simulink model "MicroMouseTemplate"  (R2023a)
settings: Solver=FixedStepAuto  StartTime=0.0  StopTime=10.0  RelTol=1e-3
values from neighbouring files (symbols this model uses):
  IR_LED_PERIOD = 0.05    [runMeFirst.m]
  signalWindowLength = 20    [runMeFirst.m]
  TIM3_ARR = 4000    [runMeFirst.m]
undefined symbols (not defined in the file or in its folder): ADC_H, ADC_L
libraries: dspstat3 x36, stm32f4xxblockslib x16, stm32l4xxblockslib x4, stm32blockslib x1
settings Model: Creator=JesseJabezArendse  LastModifiedBy=JesseJabezArendse
settings SolverCC: AllowMultiTaskInputOutput=on  InsertRTBMode=Never (minimum delay)
settings OptimizationCC: EnhancedBackFolding=on  PassReuseOutputArgsAs=Individual arguments  ZeroExternalMemoryAtStartup=off  ZeroInternalMemoryAtStartup=off  MaxStackSize=64  OptimizeBlockOrder=speed  DifferentSizesBufferReuse=on  OptimizationCustomize=off  EfficientTunableParamExpr=on
settings DebuggingCC: MultiTaskCondExecSysMsg=none  ParameterOverflowMsg=none  ParameterPrecisionLossMsg=none  ParameterTunabilityLossMsg=error
settings HardwareCC: ProdBitPerPointer=32  ProdBitPerSizeT=32  ProdBitPerPtrDiffT=32  ProdLargestAtomicInteger=Long  ProdLargestAtomicFloat=Double  ProdWordSize=32  ProdLongLongMode=on  ProdHWDeviceType=ARM Compatible->ARM Cortex
settings ModelReferenceCC: EnableParallelModelReferenceBuilds=on
settings SFSimCC: MATLABDynamicMemAlloc=off
settings RTWCC: Description=Embedded Coder  SystemTargetFile=ert.tlc  HardwareBoard=STM32L4xx Based  TemplateMakefile=ert_default_tmf  Toolchain=GNU Tools for ARM Embedded Processors
settings RTWCC: CustomHeaderCode=|
  | #include "MicroMouseProgramming\Core\Inc\IMU.h"
  | #include "MicroMouseProgramming\Core\Inc\CustomWhile.h"
  | #include "MicroMouseProgramming\Core\Inc\Motors.h"
settings RTWCC: CustomInclude=|
  | MicroMouseProgramming\Core\Inc\
  | MicroMouseProgramming\Core\Src\
settings RTWCC: CustomSource=|
  | MicroMouseProgramming\Core\Src\IMU.c
  | MicroMouseProgramming\Core\Src\CustomWhile.c
  | MicroMouseProgramming\Core\Src\Motors.c
settings CodeAppCC: ForceParamTrailComments=on  IgnoreCustomStorageClasses=off  OperatorAnnotations=on  SimulinkDataObjDesc=on  SFDataObjDesc=on  InsertBlockDesc=on
settings ERTTargetCC: CodeReplacementLibrary=ARM Cortex-M  SupportContinuousTime=on  ExtModeTransport=3  ExtModeStaticAlloc=on  ExtModeStaticAllocSize=2048  ExtModeMexFile=ext_xcp  ExtModeIntrfLevel=Level2 - Open

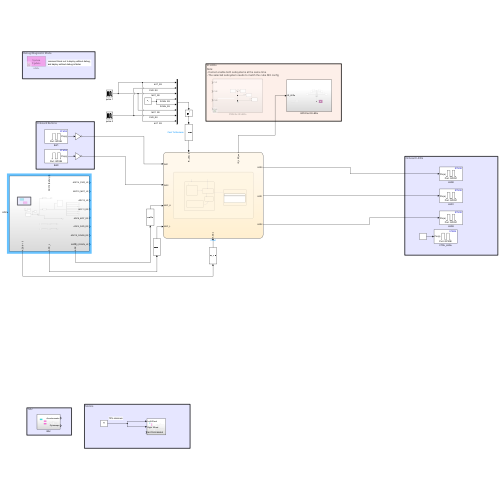
[thumbnail: Simulink's stored preview of the top-level diagram]
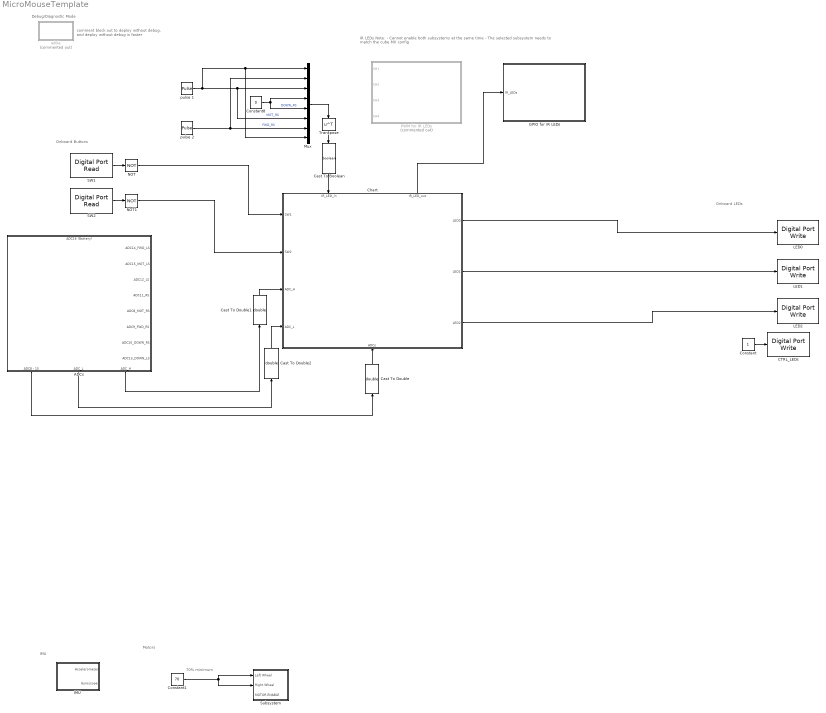
== system MicroMouseTemplate ==
  note: 70% minimum
  note: Motors
  note: IR LEDs
      | Note:
      | - Cannot enable both subsystems at the same time
      | - The selected subsystem needs to match the cube MX config
  note: IMU
  note: Onboard Buttons
  note: comment block out to deploy without debug, and deploy without debug is faster
  note: Onboard LEDs
  note: Debug/Diagnostic Mode
  "ADCs " : Subsystem
      settings: PortSchema="{\"entries\":[{\"content\":{\"sides\":[{\"content\":{},\"type\":\"ConnectorPlacement.EquallySpacedRectSide\",\"uuid\":\"ad9b4559-80f4-4a8a-ae53-5c16a02c7140\"},{\"content\":{\"connectorIds\":[\"Out1\",\"Out2\",\"Out3\",\"Out4\",\"Out5\",\"Out6\",\"Out7\",\"Out8\"],\"side\":\"RIGHT\"},\"type\":\"ConnectorPlacement.EquallySpacedRectSide\",\"uuid\":\"bb9b2394-70a2-4e95-b5de-6e9e6d3444df\"},{\"content\":{\"connectorIds\":[\"Out12\"],\"side\":\"TOP\"},\"type\":\"ConnectorPlacement.EquallySpacedRectSide\",\"uuid\":\"a0caae28-44ef-4496-b197-488b1b027954\"},{\"content\":{\"connectorIds\":[\"Out9\",\"Out10\",\"Out11\"],\"side\":\"BOTTOM\"},\"type\":\"ConnectorPlacement.EquallySpacedRectSide\",\"uuid\":\"aca5f2a6-b788-4b53-b626-f7b89ca7e1d4\"}]},\"type\":\"ConnectorPlacement.EquallySpacedConnector\",\"uuid\":\"1ade7d4f-8aae-4b0d-9bfd-23fa99654b08\"}],\"packageUris\":[\"http://schema.mathworks.com/mf0/Connector/R2020b\"],\"version\":\"1.0\"}"
  CTRL_LEDs : stm32f4xxblockslib/Digital Port Write  PortName=GPIOB  PinNumber=3  ReadOperation=off  IOAsArray=on  EnableSimPort=off
      settings: LibrarySourceBlock=stm32l4xxblockslib/Digital Port Write
  Cast To Boolean : DataTypeConversion  OutDataTypeStr=boolean  SaturateOnIntegerOverflow=off  RndMeth=Floor
  Cast To Double : DataTypeConversion  OutDataTypeStr=double  SaturateOnIntegerOverflow=off  RndMeth=Floor
  Cast To Double1 : DataTypeConversion  OutDataTypeStr=double  SaturateOnIntegerOverflow=off  RndMeth=Floor
  Cast To Double2 : DataTypeConversion  OutDataTypeStr=double  SaturateOnIntegerOverflow=off  RndMeth=Floor
  Chart : Stateflow chart  TreatAsAtomicUnit=on
      settings: PortSchema="{\"entries\":[{\"content\":{\"sides\":[{\"content\":{\"connectorIds\":[\"In2\",\"In3\",\"In4\",\"In5\"]},\"type\":\"ConnectorPlacement.EquallySpacedRectSide\",\"uuid\":\"32f6fed0-3232-4bab-b39d-a3af84b75639\"},{\"content\":{\"connectorIds\":[\"Out1\",\"Out2\",\"Out3\"],\"side\":\"RIGHT\"},\"type\":\"ConnectorPlacement.EquallySpacedRectSide\",\"uuid\":\"0c32a1fe-915a-4e8a-b3ee-800457e23572\"},{\"content\":{\"connectorIds\":[\"In6\",\"Out4\"],\"side\":\"TOP\"},\"type\":\"ConnectorPlacement.EquallySpacedRectSide\",\"uuid\":\"1ac04b60-bb97-4700-a588-8796c93b1b04\"},{\"content\":{\"connectorIds\":[\"In1\"],\"side\":\"BOTTOM\"},\"type\":\"ConnectorPlacement.EquallySpacedRectSide\",\"uuid\":\"5382ec1b-aa52-4e38-a7ba-82e952b8f427\"}]},\"type\":\"ConnectorPlacement.EquallySpacedConnector\",\"uuid\":\"e2f36b59-a9e2-4f43-a02a-04bcc2f7ebe2\"}],\"packageUris\":[\"http://schema.mathworks.com/mf0/Connector/R2020b\"],\"version\":\"1.0\"}"
  Constant : Constant
  Constant1 : Constant  Value=70
  Constant8 : Constant  Value=0
  GPIO for IR LEDs : Subsystem
  IMU : Subsystem
  LED0 : stm32f4xxblockslib/Digital Port Write  PortName=GPIOC  PinNumber=[13]  ReadOperation=off  IOAsArray=on  EnableSimPort=off
      settings: LibrarySourceBlock=stm32l4xxblockslib/Digital Port Write
  LED1 : stm32f4xxblockslib/Digital Port Write  PortName=GPIOC  PinNumber=[14]  ReadOperation=off  IOAsArray=on  EnableSimPort=off
      settings: LibrarySourceBlock=stm32l4xxblockslib/Digital Port Write
  LED2 : stm32f4xxblockslib/Digital Port Write  PortName=GPIOC  PinNumber=[15]  ReadOperation=off  IOAsArray=on  EnableSimPort=off
      settings: LibrarySourceBlock=stm32l4xxblockslib/Digital Port Write
  Mux : Mux  Inputs=8
  NOT : Logic  Operator=NOT  IconShape=distinctive  AllPortsSameDT=off  OutDataTypeStr=boolean
  NOT1 : Logic  Operator=NOT  IconShape=distinctive  AllPortsSameDT=off  OutDataTypeStr=boolean
  "PWM for IR LEDs " : Subsystem  Commented=on
  SW1 : stm32f4xxblockslib/Digital Port Read  PortName=GPIOE  PinNumber=[6]  ReadOperation=on  IOAsArray=on  SampleTime=-1  EnableSimPort=off
      settings: LibrarySourceBlock=stm32l4xxblockslib/Digital Port Read
  SW2 : stm32f4xxblockslib/Digital Port Read  PortName=GPIOB  PinNumber=[2]  ReadOperation=on  IOAsArray=on  SampleTime=-1  EnableSimPort=off
      settings: LibrarySourceBlock=stm32l4xxblockslib/Digital Port Read
  Subsystem : Subsystem
  Transpose : Math  Operator=transpose
  pulse 1 : DiscretePulseGenerator  PulseType=Time based  Period=3*IR_LED_PERIOD  PulseWidth=1/4*100
  pulse 2 : DiscretePulseGenerator  PulseType=Time based  Period=3*IR_LED_PERIOD  PulseWidth=1/4*100  PhaseDelay=2*IR_LED_PERIOD
  while : Subsystem  Commented=on  mask(System Update){ShowInLibBrowser=0}
      mask prompts: ShowInLibBrowser "Simulink:masks:CustCodeMaskParam1_MP"
      settings: CopyFcn=cccopyfcn(gcb)  OpenFcn=ccopenfcn('System Update Function')
      mask Help: eval('feval(''rtwprivate'',''rtwhelpview'',''rtw_sys_update_block'')');
      mask DialogControl ShowInLibBrowser Prompt: Mask Parameter 1:
      mask Display: disp('System\nUpdate');
  wires:
  SW2/1 -> NOT1/1
  Constant/1 -> CTRL_LEDs/1
  SW1/1 -> NOT/1
  Constant1/1 -> Subsystem/1(Left Wheel), Subsystem/2(Right Wheel)
  pulse 2/1 -> Mux/2, Mux/7  "FWD_RS"
  pulse 1/1 -> Mux/8, Mux/1, Mux/6, Mux/3  "MOT_RS"
  Constant8/1 -> Mux/4, Mux/5  "DOWN_RS"
  Mux/1 -> Transpose/1
  Chart/1(LED0) -> LED0/1
  Chart/2(LED1) -> LED1/1
  Chart/3(LED2) -> LED2/1
  "ADCs "/11(ADC_H) -> Cast To Double1/1
  "ADCs "/10(ADC_L) -> Cast To Double2/1
  Chart/4(IR_LED_out) -> GPIO for IR LEDs/1(IR_LEDs)
  NOT/1 -> Chart/2(SW1)
  NOT1/1 -> Chart/3(SW2)
  Transpose/1 -> Cast To Boolean/1
  Cast To Boolean/1 -> Chart/6(IR_LED_in)
  "ADCs "/9(ADC8 - 15) -> Cast To Double/1
  Cast To Double/1 -> Chart/1(ADCs)
  Cast To Double1/1 -> Chart/4(ADC_H)
  Cast To Double2/1 -> Chart/5(ADC_L)

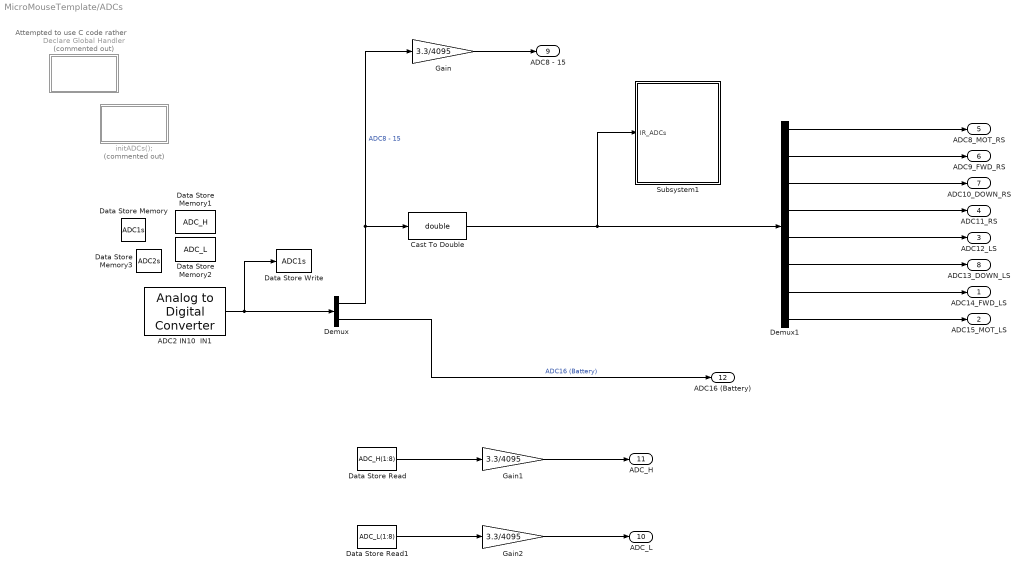
== system MicroMouseTemplate/ADCs  ==
  note: Attempted to use C code rather
  ADC2 IN10  IN1 : stm32f4xxblockslib/Analog to Digital Converter  ADCModule=ADC2  ConversionGroup=Regular  TriggerMode=Trigger and read  NumberOfConversions=9  EnableBufferConv=on  BufferLength=9  OutputStatus=off  SampleTime=-1  EnableSimPort=off
      settings: LibrarySourceBlock=stm32l4xxblockslib/Analog to Digital Converter
  Cast To Double : DataTypeConversion  OutDataTypeStr=double  SaturateOnIntegerOverflow=off  RndMeth=Floor
  Data Store Memory : DataStoreMemory  DataStoreName=ADC1s  WriteAfterWriteMsg=warning  ShowAdditionalParam=off  OutDataTypeStr=uint16  Dimensions=9
  Data Store Memory1 : DataStoreMemory  DataStoreName=ADC_H  WriteAfterWriteMsg=warning  ShowAdditionalParam=off  OutDataTypeStr=uint16  Dimensions=9
  Data Store Memory2 : DataStoreMemory  DataStoreName=ADC_L  WriteAfterWriteMsg=warning  ShowAdditionalParam=off  OutDataTypeStr=uint16  Dimensions=9
  Data Store Memory3 : DataStoreMemory  DataStoreName=ADC2s  WriteAfterWriteMsg=warning  ShowAdditionalParam=off  OutDataTypeStr=uint16  Dimensions=9
  Data Store Read : DataStoreRead  DataStoreName=ADC_H  DataStoreElements=ADC_H(1:8)  NumberOfDimensions=8  IndexOptions=Index vector (dialog),Index vector (dialog),Index vector (dialog),Index vector (dialog),Index vector (dialog),Index vector (dialog),Index vector (dialog),Index vector (dialog)  Indices=1,1,1,1,1,1,1,1  OutputSizes=1,1,1,1,1,1,1,1
  Data Store Read1 : DataStoreRead  DataStoreName=ADC_L  DataStoreElements=ADC_L(1:8)  IndexOptions=Index vector (dialog)  Indices=1  OutputSizes=1
  Data Store Write : DataStoreWrite  DataStoreName=ADC1s  IndexOptions=Index vector (dialog)  Indices=1  OutputSizes=1
  Declare Global Handler : Subsystem  Commented=on  mask(Model Source){ShowInLibBrowser=0}
      mask prompts: ShowInLibBrowser "Simulink:masks:CustCodeMaskParam1_MP"
      settings: CopyFcn=cccopyfcn(gcb)  OpenFcn=ccopenfcn('Model Source')
      mask Help: eval('feval(''rtwprivate'',''rtwhelpview'',''rtw_model_source_block'')');
      mask Display: disp('Model\nSource');
  Demux : Demux  Outputs=[8 1]
  Demux1 : Demux  Outputs=8
  Gain : Gain  Gain=3.3/4095
  Gain1 : Gain  Gain=3.3/4095
  Gain2 : Gain  Gain=3.3/4095
  Subsystem1 : Subsystem
  initADCs(); : Subsystem  Commented=on  mask(System Initialize){ShowInLibBrowser=0}
      mask prompts: ShowInLibBrowser "Simulink:masks:CustCodeMaskParam1_MP"
      settings: CopyFcn=cccopyfcn(gcb)  OpenFcn=ccopenfcn('System Initialize Function')
      mask Help: eval('feval(''rtwprivate'',''rtwhelpview'',''rtw_sys_initialize_block'')');
      mask Display: disp('System\nInitialize');
  ADC14_FWD_LS : Outport
  ADC15_MOT_LS : Outport  Port=2
  ADC12_LS : Outport  Port=3
  ADC11_RS : Outport  Port=4
  ADC8_MOT_RS : Outport  Port=5
  ADC9_FWD_RS : Outport  Port=6
  ADC10_DOWN_RS : Outport  Port=7
  ADC13_DOWN_LS : Outport  Port=8
  ADC8 - 15 : Outport  Port=9
  ADC_L : Outport  Port=10
  ADC_H : Outport  Port=11
  ADC16 (Battery) : Outport  Port=12
  wires:
  Demux/1 -> Gain/1, Cast To Double/1  "ADC8 - 15"
  Demux/2 -> ADC16 (Battery)/1  "ADC16 (Battery)"
  Demux1/1 -> ADC8_MOT_RS/1
  Demux1/2 -> ADC9_FWD_RS/1
  Demux1/3 -> ADC10_DOWN_RS/1
  Demux1/4 -> ADC11_RS/1
  Demux1/5 -> ADC12_LS/1
  Demux1/6 -> ADC13_DOWN_LS/1
  Demux1/7 -> ADC14_FWD_LS/1
  Demux1/8 -> ADC15_MOT_LS/1
  ADC2 IN10  IN1/1 -> Data Store Write/1, Demux/1
  Cast To Double/1 -> Demux1/1, Subsystem1/1(IR_ADCs)
  Gain/1 -> ADC8 - 15/1
  Data Store Read/1 -> Gain1/1
  Data Store Read1/1 -> Gain2/1
  Gain1/1 -> ADC_H/1
  Gain2/1 -> ADC_L/1

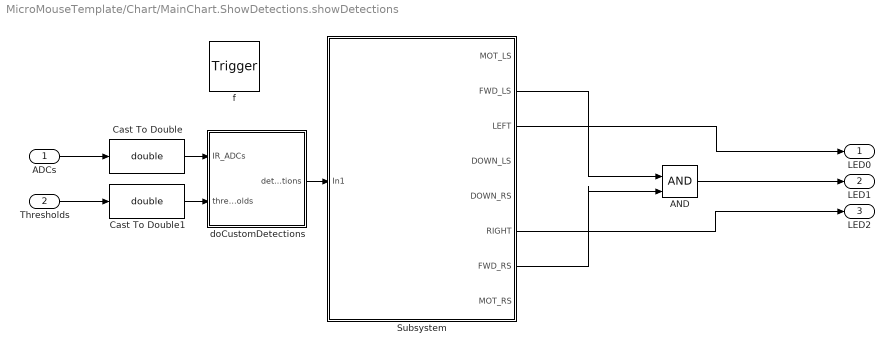
== system MicroMouseTemplate/Chart/MainChart.ShowDetections.showDetections ==
  ADCs : Inport  OutDataTypeStr=double  PortDimensions=8
  Thresholds : Inport  Port=2  OutDataTypeStr=double  PortDimensions=8
  f : TriggerPort  TriggerType=function-call  VariantControl=(inherit)
      settings: CopyFcn=Stateflow.SLINSF.SimulinkMan.removeBlockPreDeleteFcn  PreDeleteFcn=Stateflow.SLINSF.SimulinkMan.unsafePredeleteFcn
  AND : Logic  IconShape=distinctive  AllPortsSameDT=off  OutDataTypeStr=boolean
  Cast To Double : DataTypeConversion  OutDataTypeStr=double  SaturateOnIntegerOverflow=off  RndMeth=Floor
  Cast To Double1 : DataTypeConversion  OutDataTypeStr=double  SaturateOnIntegerOverflow=off  RndMeth=Floor
  Subsystem : Subsystem
  doCustomDetections : Subsystem
  LED0 : Outport
  LED1 : Outport  Port=2
  LED2 : Outport  Port=3
  wires:
  Subsystem/7(FWD_RS) -> AND/2
  AND/1 -> LED1/1
  Subsystem/2(FWD_LS) -> AND/1
  Subsystem/3(LEFT) -> LED0/1
  Subsystem/6(RIGHT) -> LED2/1
  ADCs/1 -> Cast To Double/1
  Thresholds/1 -> Cast To Double1/1
  doCustomDetections/1(detections) -> Subsystem/1(In1)
  Cast To Double/1 -> doCustomDetections/1(IR_ADCs)
  Cast To Double1/1 -> doCustomDetections/2(thresholds)

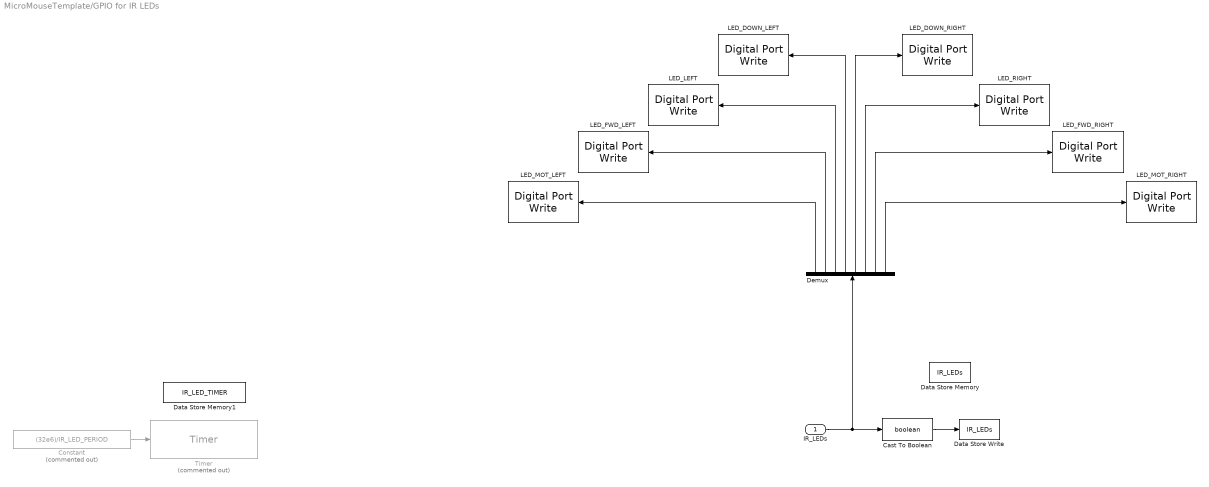
== system MicroMouseTemplate/GPIO for IR LEDs ==
  IR_LEDs : Inport
  Cast To Boolean : DataTypeConversion  OutDataTypeStr=boolean  SaturateOnIntegerOverflow=off  RndMeth=Floor
  Constant : Constant  Commented=on  Value=(32e6)/IR_LED_PERIOD
  Data Store Memory : DataStoreMemory  DataStoreName=IR_LEDs  WriteAfterWriteMsg=warning  ShowAdditionalParam=off  OutDataTypeStr=boolean  Dimensions=8
  Data Store Memory1 : DataStoreMemory  DataStoreName=IR_LED_TIMER  WriteAfterWriteMsg=warning  ShowAdditionalParam=off  OutDataTypeStr=uint32  Dimensions=1
  Data Store Write : DataStoreWrite  DataStoreName=IR_LEDs  IndexOptions=Index vector (dialog)  Indices=1  OutputSizes=1
  Demux : Demux  Outputs=8
  LED_DOWN_LEFT : stm32f4xxblockslib/Digital Port Write  PortName=GPIOE  PinNumber=9  ReadOperation=off  IOAsArray=on  EnableSimPort=off
      settings: LibrarySourceBlock=stm32l4xxblockslib/Digital Port Write
  LED_DOWN_RIGHT : stm32f4xxblockslib/Digital Port Write  PortName=GPIOE  PinNumber=14  ReadOperation=off  IOAsArray=on  EnableSimPort=off
      settings: LibrarySourceBlock=stm32l4xxblockslib/Digital Port Write
  LED_FWD_LEFT : stm32f4xxblockslib/Digital Port Write  PortName=GPIOE  PinNumber=8  ReadOperation=off  IOAsArray=on  EnableSimPort=off
      settings: LibrarySourceBlock=stm32l4xxblockslib/Digital Port Write
  LED_FWD_RIGHT : stm32f4xxblockslib/Digital Port Write  PortName=GPIOE  PinNumber=15  ReadOperation=off  IOAsArray=on  EnableSimPort=off
      settings: LibrarySourceBlock=stm32l4xxblockslib/Digital Port Write
  LED_LEFT : stm32f4xxblockslib/Digital Port Write  PortName=GPIOE  PinNumber=12  ReadOperation=off  IOAsArray=on  EnableSimPort=off
      settings: LibrarySourceBlock=stm32l4xxblockslib/Digital Port Write
  LED_MOT_LEFT : stm32f4xxblockslib/Digital Port Write  PortName=GPIOB  PinNumber=12  ReadOperation=off  IOAsArray=on  EnableSimPort=off
      settings: LibrarySourceBlock=stm32l4xxblockslib/Digital Port Write
  LED_MOT_RIGHT : stm32f4xxblockslib/Digital Port Write  PortName=GPIOE  PinNumber=13  ReadOperation=off  IOAsArray=on  EnableSimPort=off
      settings: LibrarySourceBlock=stm32l4xxblockslib/Digital Port Write
  LED_RIGHT : stm32f4xxblockslib/Digital Port Write  PortName=GPIOE  PinNumber=11  ReadOperation=off  IOAsArray=on  EnableSimPort=off
      settings: LibrarySourceBlock=stm32l4xxblockslib/Digital Port Write
  Timer : stm32blockslib/Timer  Priority=4  Commented=on  TimerModule=TIM4  EnableFrequencyInput=on  EnableCounterInput=off  EnableMainOutputInput=off  SetRCAfterCE=off  OutputDirection=off  OutputMainOutputEnableStatus=off  SampleTime=-1  EnableUpdateEvent=off  EnableCaptureCompare1Event=off  EnableCaptureCompare2Event=off  EnableCaptureCompare3Event=off  EnableCaptureCompare4Event=off  EnableTriggerEvent=off  EnableBreakEvent=off  EnableBreakEvent2=off  EnableCOMGenerationEvent=off  ProcessorFamily=STM32L4
      settings: LibrarySourceBlock=stm32l4xxblockslib/Timer
  wires:
  Demux/1 -> LED_MOT_LEFT/1
  Demux/2 -> LED_FWD_LEFT/1
  Demux/3 -> LED_LEFT/1
  Constant/1 -> Timer/1
  IR_LEDs/1 -> Demux/1, Cast To Boolean/1
  Demux/6 -> LED_RIGHT/1
  Demux/7 -> LED_FWD_RIGHT/1
  Demux/8 -> LED_MOT_RIGHT/1
  Demux/4 -> LED_DOWN_LEFT/1
  Demux/5 -> LED_DOWN_RIGHT/1
  Cast To Boolean/1 -> Data Store Write/1

== system MicroMouseTemplate/IMU ==
  Data Store Memory : DataStoreMemory  DataStoreName=IMU_Accel  WriteAfterWriteMsg=warning  ShowAdditionalParam=off  OutDataTypeStr=single  Dimensions=3
  Data Store Memory1 : DataStoreMemory  DataStoreName=IMU_Gyro  WriteAfterWriteMsg=warning  ShowAdditionalParam=off  OutDataTypeStr=single  Dimensions=3
  Data Store Read : DataStoreRead  DataStoreName=IMU_Accel  IndexOptions=Index vector (dialog)  Indices=1  OutputSizes=1
  Data Store Read1 : DataStoreRead  DataStoreName=IMU_Gyro  IndexOptions=Index vector (dialog)  Indices=1  OutputSizes=1
  Declare Global Handler : Subsystem  mask(Model Source){ShowInLibBrowser=0}
      mask prompts: ShowInLibBrowser "Simulink:masks:CustCodeMaskParam1_MP"
      settings: CopyFcn=cccopyfcn(gcb)  OpenFcn=ccopenfcn('Model Source')
      mask Help: eval('feval(''rtwprivate'',''rtwhelpview'',''rtw_model_source_block'')');
      mask Display: disp('Model\nSource');
  initIMU(); : Subsystem  mask(System Initialize){ShowInLibBrowser=0}
      mask prompts: ShowInLibBrowser "Simulink:masks:CustCodeMaskParam1_MP"
      settings: CopyFcn=cccopyfcn(gcb)  OpenFcn=ccopenfcn('System Initialize Function')
      mask Help: eval('feval(''rtwprivate'',''rtwhelpview'',''rtw_sys_initialize_block'')');
      mask Display: disp('System\nInitialize');
  refreshIMUValues(); : Subsystem  mask(System Update){ShowInLibBrowser=0}
      mask prompts: ShowInLibBrowser "Simulink:masks:CustCodeMaskParam1_MP"
      settings: CopyFcn=cccopyfcn(gcb)  OpenFcn=ccopenfcn('System Update Function')
      mask Help: eval('feval(''rtwprivate'',''rtwhelpview'',''rtw_sys_update_block'')');
      mask Display: disp('System\nUpdate');
  Accelerometer : Outport
  Gyroscope : Outport  Port=2
  wires:
  Data Store Read1/1 -> Gyroscope/1
  Data Store Read/1 -> Accelerometer/1

== system MicroMouseTemplate/PWM for IR LEDs  ==
  note: the others are not availible, either a negative channel or not a PWM pin
  CH1 : Inport
  CH2 : Inport  Port=2
  CH3 : Inport  Port=3
  CH4 : Inport  Port=4
  ENABLE PWM MODE : Constant  Value=0
  LED_PWM_FWD_RIGHT : stm32l4xxblockslib/PWM Output  TimerModule=TIM1  DutycycleUnits=Percentage  EnableChannel1=off  EnableChannel2=off  EnableChannel3=on  EnableChannel4=off  EnableChannel5=off  EnableChannel6=off  EnableCounterInput=on  EnableMainOutputInput=off  EnableFrequencyInput=off  SetRCAfterCE=off  OutputDirection=off  OutputMainOutputEnableStatus=off  SampleTime=0.1  EnableSimPort=off  EnableUpdateEvent=off  EnableCaptureCompare1Event=off  EnableCaptureCompare2Event=off  EnableCaptureCompare3Event=off  EnableCaptureCompare4Event=off  EnableTriggerEvent=off  EnableBreakEvent=off  EnableBreakEvent2=off  ProcessorFamily=STM32L4  hoistedMaskSrc=ECSoC/ECSimCodegen/PWM Output
  LED_PWM_LEFT : stm32l4xxblockslib/PWM Output  TimerModule=TIM1  DutycycleUnits=Percentage  EnableChannel1=on  EnableChannel2=off  EnableChannel3=off  EnableChannel4=off  EnableChannel5=off  EnableChannel6=off  EnableCounterInput=on  EnableMainOutputInput=off  EnableFrequencyInput=off  SetRCAfterCE=off  OutputDirection=off  OutputMainOutputEnableStatus=off  SampleTime=0.1  EnableSimPort=off  EnableUpdateEvent=off  EnableCaptureCompare1Event=off  EnableCaptureCompare2Event=off  EnableCaptureCompare3Event=off  EnableCaptureCompare4Event=off  EnableTriggerEvent=off  EnableBreakEvent=off  EnableBreakEvent2=off  ProcessorFamily=STM32L4  hoistedMaskSrc=ECSoC/ECSimCodegen/PWM Output
  LED_PWM_MOT_RIGHT : stm32l4xxblockslib/PWM Output  TimerModule=TIM17  DutycycleUnits=Percentage  EnableChannel1=on  EnableChannel2=off  EnableChannel3=off  EnableChannel4=off  EnableChannel5=off  EnableChannel6=off  EnableCounterInput=on  EnableMainOutputInput=off  EnableFrequencyInput=off  SetRCAfterCE=off  OutputDirection=off  OutputMainOutputEnableStatus=off  SampleTime=0.1  EnableSimPort=off  EnableUpdateEvent=off  EnableCaptureCompare1Event=off  EnableCaptureCompare2Event=off  EnableCaptureCompare3Event=off  EnableCaptureCompare4Event=off  EnableTriggerEvent=off  EnableBreakEvent=off  EnableBreakEvent2=off  ProcessorFamily=STM32L4  hoistedMaskSrc=ECSoC/ECSimCodegen/PWM Output
  LED_PWM_RIGHT : stm32l4xxblockslib/PWM Output  TimerModule=TIM1  DutycycleUnits=Percentage  EnableChannel1=off  EnableChannel2=on  EnableChannel3=off  EnableChannel4=off  EnableChannel5=off  EnableChannel6=off  EnableCounterInput=on  EnableMainOutputInput=off  EnableFrequencyInput=off  SetRCAfterCE=off  OutputDirection=off  OutputMainOutputEnableStatus=off  SampleTime=0.1  EnableSimPort=off  EnableUpdateEvent=off  EnableCaptureCompare1Event=off  EnableCaptureCompare2Event=off  EnableCaptureCompare3Event=off  EnableCaptureCompare4Event=off  EnableTriggerEvent=off  EnableBreakEvent=off  EnableBreakEvent2=off  ProcessorFamily=STM32L4  hoistedMaskSrc=ECSoC/ECSimCodegen/PWM Output
  wires:
  ENABLE PWM MODE/1 -> LED_PWM_RIGHT/2, LED_PWM_LEFT/2, LED_PWM_FWD_RIGHT/2, LED_PWM_MOT_RIGHT/2
  CH1/1 -> LED_PWM_LEFT/1
  CH4/1 -> LED_PWM_MOT_RIGHT/1
  CH2/1 -> LED_PWM_RIGHT/1
  CH3/1 -> LED_PWM_FWD_RIGHT/1

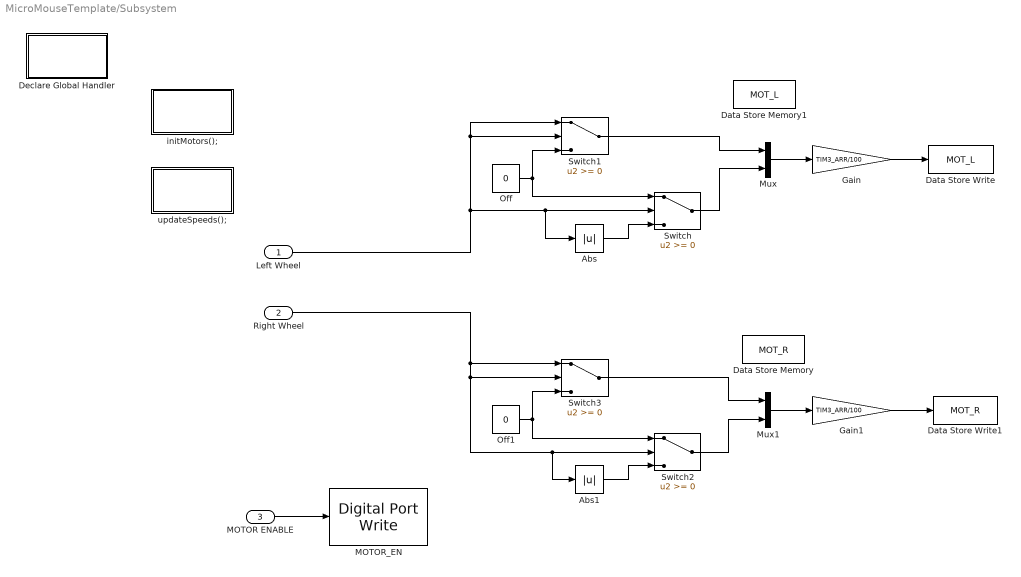
== system MicroMouseTemplate/Subsystem ==
  Left Wheel : Inport
  Right Wheel : Inport  Port=2
  MOTOR ENABLE : Inport  Port=3
  Abs : Abs  SaturateOnIntegerOverflow=off
  Abs1 : Abs  SaturateOnIntegerOverflow=off
  Data Store Memory : DataStoreMemory  DataStoreName=MOT_R  WriteAfterWriteMsg=warning  ShowAdditionalParam=off  OutDataTypeStr=uint16  Dimensions=2
  Data Store Memory1 : DataStoreMemory  DataStoreName=MOT_L  WriteAfterWriteMsg=warning  ShowAdditionalParam=off  OutDataTypeStr=uint16  Dimensions=2
  Data Store Write : DataStoreWrite  DataStoreName=MOT_L  IndexOptions=Index vector (dialog)  Indices=1  OutputSizes=1
  Data Store Write1 : DataStoreWrite  DataStoreName=MOT_R  IndexOptions=Index vector (dialog)  Indices=1  OutputSizes=1
  Declare Global Handler : Subsystem  mask(Model Source){ShowInLibBrowser=0}
      mask prompts: ShowInLibBrowser "Simulink:masks:CustCodeMaskParam1_MP"
      settings: CopyFcn=cccopyfcn(gcb)  OpenFcn=ccopenfcn('Model Source')
      mask Help: eval('feval(''rtwprivate'',''rtwhelpview'',''rtw_model_source_block'')');
      mask Display: disp('Model\nSource');
  Gain : Gain  Gain=TIM3_ARR/100  OutDataTypeStr=uint16
  Gain1 : Gain  Gain=TIM3_ARR/100  OutDataTypeStr=uint16
  MOTOR_EN : stm32f4xxblockslib/Digital Port Write  PortName=GPIOD  PinNumber=7  ReadOperation=off  IOAsArray=on  EnableSimPort=off
      settings: LibrarySourceBlock=stm32l4xxblockslib/Digital Port Write
  Mux : Mux  Inputs=2
  Mux1 : Mux  Inputs=2
  Off : Constant  Value=0
  Off1 : Constant  Value=0
  Switch{,1..3} (4 alike) : Switch  SaturateOnIntegerOverflow=off  InputSameDT=off
  initMotors(); : Subsystem  mask(System Initialize){ShowInLibBrowser=0}
      mask prompts: ShowInLibBrowser "Simulink:masks:CustCodeMaskParam1_MP"
      settings: CopyFcn=cccopyfcn(gcb)  OpenFcn=ccopenfcn('System Initialize Function')
      mask Help: eval('feval(''rtwprivate'',''rtwhelpview'',''rtw_sys_initialize_block'')');
      mask Display: disp('System\nInitialize');
  updateSpeeds(); : Subsystem  mask(System Update){ShowInLibBrowser=0}
      mask prompts: ShowInLibBrowser "Simulink:masks:CustCodeMaskParam1_MP"
      settings: CopyFcn=cccopyfcn(gcb)  OpenFcn=ccopenfcn('System Update Function')
      mask Help: eval('feval(''rtwprivate'',''rtwhelpview'',''rtw_sys_update_block'')');
      mask Display: disp('System\nUpdate');
  wires:
  Abs1/1 -> Switch2/3
  Switch1/1 -> Mux/1
  Off/1 -> Switch/1, Switch1/3
  Off1/1 -> Switch2/1, Switch3/3
  Switch/1 -> Mux/2
  Switch3/1 -> Mux1/1
  Abs/1 -> Switch/3
  Switch2/1 -> Mux1/2
  MOTOR ENABLE/1 -> MOTOR_EN/1
  Left Wheel/1 -> Abs/1, Switch/2, Switch1/2, Switch1/1
  Right Wheel/1 -> Switch3/2, Switch2/2, Abs1/1, Switch3/1
  Mux/1 -> Gain/1
  Mux1/1 -> Gain1/1
  Gain1/1 -> Data Store Write1/1
  Gain/1 -> Data Store Write/1

== system MicroMouseTemplate/while ==

== system MicroMouseTemplate/ADCs /Declare Global Handler ==

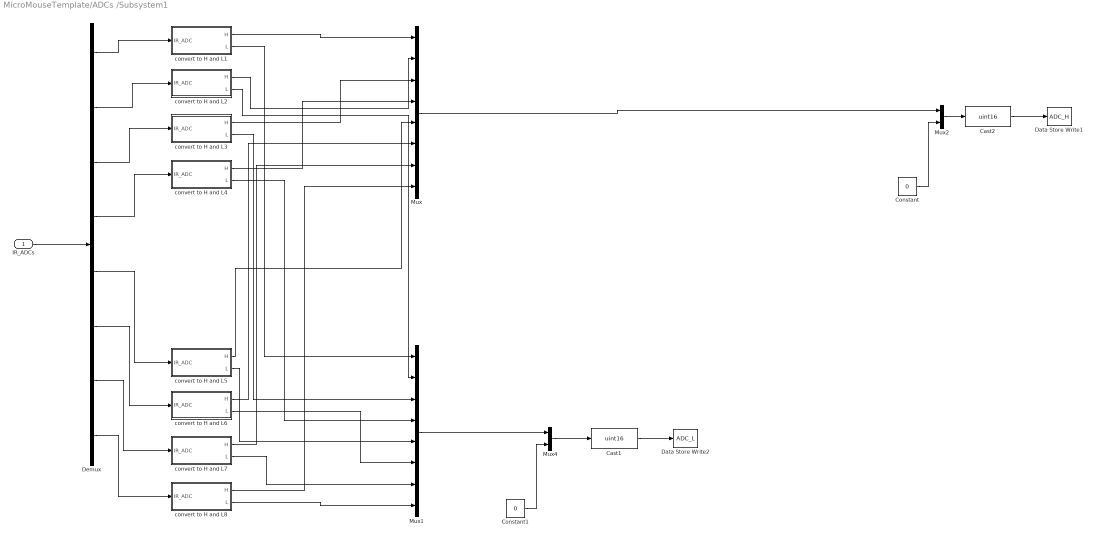
== system MicroMouseTemplate/ADCs /Subsystem1 ==
  IR_ADCs : Inport
  Cast1 : DataTypeConversion  OutDataTypeStr=uint16  SaturateOnIntegerOverflow=off  RndMeth=Floor
  Cast2 : DataTypeConversion  OutDataTypeStr=uint16  SaturateOnIntegerOverflow=off  RndMeth=Floor
  Constant : Constant  Value=0
  Constant1 : Constant  Value=0
  Data Store Write1 : DataStoreWrite  DataStoreName=ADC_H  IndexOptions=Index vector (dialog)  Indices=1  OutputSizes=1
  Data Store Write2 : DataStoreWrite  DataStoreName=ADC_L  IndexOptions=Index vector (dialog)  Indices=1  OutputSizes=1
  Demux : Demux  Outputs=8
  Mux : Mux  Inputs=8
  Mux1 : Mux  Inputs=8
  Mux2 : Mux  Inputs=2
  Mux4 : Mux  Inputs=2
  convert to H and L1 : Subsystem
  convert to H and L2 : Subsystem
  convert to H and L3 : Subsystem
  convert to H and L4 : Subsystem
  convert to H and L5 : Subsystem
  convert to H and L6 : Subsystem
  convert to H and L7 : Subsystem
  convert to H and L8 : Subsystem
  wires:
  convert to H and L8/2(L) -> Mux1/8
  Demux/3 -> convert to H and L3/1(IR_ADC)
  Demux/4 -> convert to H and L4/1(IR_ADC)
  Demux/8 -> convert to H and L8/1(IR_ADC)
  convert to H and L8/1(H) -> Mux/8
  Demux/1 -> convert to H and L1/1(IR_ADC)
  Demux/7 -> convert to H and L7/1(IR_ADC)
  Demux/2 -> convert to H and L2/1(IR_ADC)
  Demux/5 -> convert to H and L5/1(IR_ADC)
  Demux/6 -> convert to H and L6/1(IR_ADC)
  convert to H and L1/1(H) -> Mux/1
  convert to H and L7/1(H) -> Mux/7
  convert to H and L1/2(L) -> Mux1/1
  convert to H and L2/1(H) -> Mux/2
  convert to H and L2/2(L) -> Mux1/2
  convert to H and L3/1(H) -> Mux/3
  convert to H and L7/2(L) -> Mux1/7
  convert to H and L3/2(L) -> Mux1/3
  convert to H and L4/1(H) -> Mux/4
  convert to H and L4/2(L) -> Mux1/4
  convert to H and L5/1(H) -> Mux/5
  convert to H and L5/2(L) -> Mux1/5
  convert to H and L6/1(H) -> Mux/6
  convert to H and L6/2(L) -> Mux1/6
  IR_ADCs/1 -> Demux/1
  Mux2/1 -> Cast2/1
  Constant/1 -> Mux2/2
  Mux/1 -> Mux2/1
  Constant1/1 -> Mux4/2
  Mux1/1 -> Mux4/1
  Mux4/1 -> Cast1/1
  Cast2/1 -> Data Store Write1/1
  Cast1/1 -> Data Store Write2/1

== system MicroMouseTemplate/ADCs /initADCs(); ==

== system MicroMouseTemplate/Chart/MainChart.ShowDetections.showDetections/Subsystem ==
  In1 : Inport
  Demux2 : Demux  Outputs=8
  MOT_LS : Outport
  FWD_LS : Outport  Port=2
  LEFT : Outport  Port=3
  DOWN_LS : Outport  Port=4
  DOWN_RS : Outport  Port=5
  RIGHT : Outport  Port=6
  FWD_RS : Outport  Port=7
  MOT_RS : Outport  Port=8
  wires:
  In1/1 -> Demux2/1
  Demux2/2 -> FWD_RS/1  "FWD_RS"
  Demux2/1 -> MOT_RS/1  "MOT_RS"
  Demux2/5 -> LEFT/1  "LEFT"
  Demux2/4 -> RIGHT/1  "RIGHT"
  Demux2/6 -> DOWN_LS/1  "DOWN_LS"
  Demux2/3 -> DOWN_RS/1  "DOWN_RS"
  Demux2/8 -> MOT_LS/1  "MOT_LS"
  Demux2/7 -> FWD_LS/1  "FWD_LS"

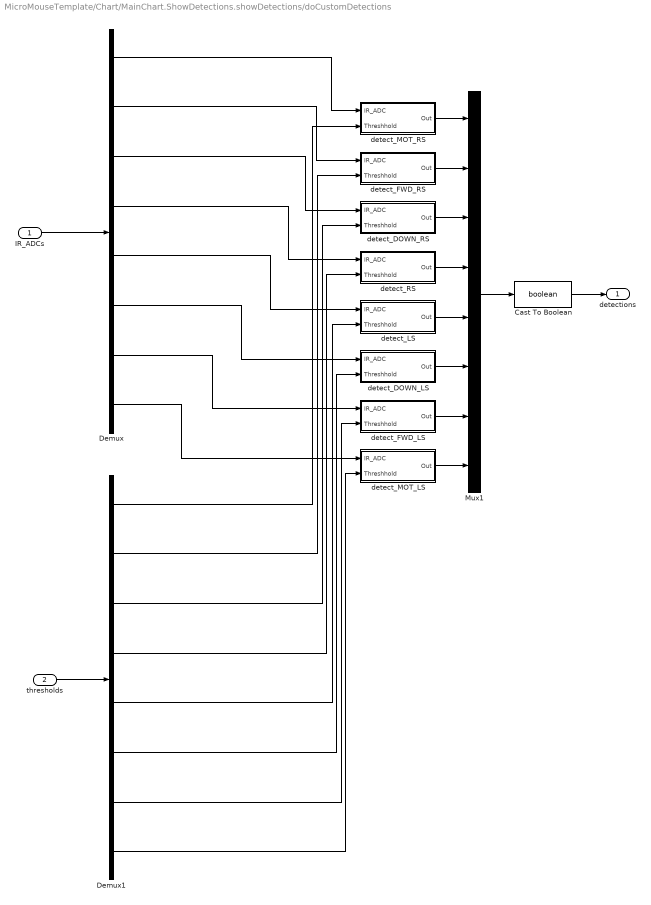
== system MicroMouseTemplate/Chart/MainChart.ShowDetections.showDetections/doCustomDetections ==
  IR_ADCs : Inport
  thresholds : Inport  Port=2
  Cast To Boolean : DataTypeConversion  OutDataTypeStr=boolean  SaturateOnIntegerOverflow=off  RndMeth=Floor
  Demux : Demux  Outputs=8
  Demux1 : Demux  Outputs=8
  Mux1 : Mux  Inputs=8
  detect_DOWN_LS : Subsystem
  detect_DOWN_RS : Subsystem
  detect_FWD_LS : Subsystem
  detect_FWD_RS : Subsystem
  detect_LS : Subsystem
  detect_MOT_LS : Subsystem
  detect_MOT_RS : Subsystem
  detect_RS : Subsystem
  detections : Outport
  wires:
  Demux/8 -> detect_MOT_LS/1(IR_ADC)
  Demux/1 -> detect_MOT_RS/1(IR_ADC)
  Demux/2 -> detect_FWD_RS/1(IR_ADC)
  detect_RS/1(Out) -> Mux1/4
  thresholds/1 -> Demux1/1
  Demux1/1 -> detect_MOT_RS/2(Threshhold)
  IR_ADCs/1 -> Demux/1
  detect_MOT_RS/1(Out) -> Mux1/1
  Demux/6 -> detect_DOWN_LS/1(IR_ADC)
  Demux1/3 -> detect_DOWN_RS/2(Threshhold)
  Demux1/7 -> detect_FWD_LS/2(Threshhold)
  Demux/4 -> detect_RS/1(IR_ADC)
  Demux1/6 -> detect_DOWN_LS/2(Threshhold)
  detect_FWD_RS/1(Out) -> Mux1/2
  Demux1/2 -> detect_FWD_RS/2(Threshhold)
  Demux1/4 -> detect_RS/2(Threshhold)
  Demux1/5 -> detect_LS/2(Threshhold)
  Demux1/8 -> detect_MOT_LS/2(Threshhold)
  detect_FWD_LS/1(Out) -> Mux1/7
  Mux1/1 -> Cast To Boolean/1
  detect_DOWN_RS/1(Out) -> Mux1/3
  detect_MOT_LS/1(Out) -> Mux1/8
  detect_DOWN_LS/1(Out) -> Mux1/6
  Demux/5 -> detect_LS/1(IR_ADC)
  detect_LS/1(Out) -> Mux1/5
  Demux/7 -> detect_FWD_LS/1(IR_ADC)
  Demux/3 -> detect_DOWN_RS/1(IR_ADC)
  Cast To Boolean/1 -> detections/1

== system MicroMouseTemplate/IMU/Declare Global Handler ==

== system MicroMouseTemplate/IMU/initIMU(); ==

== system MicroMouseTemplate/IMU/refreshIMUValues(); ==

== system MicroMouseTemplate/Subsystem/Declare Global Handler ==

== system MicroMouseTemplate/Subsystem/initMotors(); ==

== system MicroMouseTemplate/Subsystem/updateSpeeds(); ==

== system MicroMouseTemplate/ADCs /Subsystem1/convert to H and L1 ==
  IR_ADC : Inport
  Moving Maximum : dspstat3/Moving Maximum  SpecifyWindowLength=on  WindowLength=signalWindowLength  SimulateUsing=Code generation
  Moving Minimum : dspstat3/Moving Minimum  SpecifyWindowLength=on  WindowLength=signalWindowLength  SimulateUsing=Code generation
  H : Outport
  L : Outport  Port=2
  wires:
  Moving Minimum/1 -> L/1
  IR_ADC/1 -> Moving Minimum/1, Moving Maximum/1
  Moving Maximum/1 -> H/1

== system MicroMouseTemplate/ADCs /Subsystem1/convert to H and L2 ==
  IR_ADC : Inport
  Moving Maximum1 : dspstat3/Moving Maximum  SpecifyWindowLength=on  WindowLength=signalWindowLength-15  SimulateUsing=Code generation
  Moving Minimum : dspstat3/Moving Minimum  SpecifyWindowLength=on  WindowLength=signalWindowLength  SimulateUsing=Code generation
  Moving Minimum2 : dspstat3/Moving Minimum  SpecifyWindowLength=on  WindowLength=signalWindowLength-5  SimulateUsing=Code generation
  H : Outport
  L : Outport  Port=2
  wires:
  Moving Minimum/1 -> L/1
  IR_ADC/1 -> Moving Maximum1/1, Moving Minimum/1
  Moving Maximum1/1 -> Moving Minimum2/1
  Moving Minimum2/1 -> H/1

== system MicroMouseTemplate/ADCs /Subsystem1/convert to H and L3 ==
  IR_ADC : Inport
  Moving Maximum : dspstat3/Moving Maximum  SpecifyWindowLength=on  WindowLength=signalWindowLength  SimulateUsing=Code generation
  Moving Minimum : dspstat3/Moving Minimum  SpecifyWindowLength=on  WindowLength=signalWindowLength  SimulateUsing=Code generation
  H : Outport
  L : Outport  Port=2
  wires:
  Moving Minimum/1 -> L/1
  Moving Maximum/1 -> H/1
  IR_ADC/1 -> Moving Minimum/1, Moving Maximum/1

== system MicroMouseTemplate/ADCs /Subsystem1/convert to H and L4 ==
  IR_ADC : Inport
  Moving Maximum : dspstat3/Moving Maximum  SpecifyWindowLength=on  WindowLength=signalWindowLength  SimulateUsing=Code generation
  Moving Minimum : dspstat3/Moving Minimum  SpecifyWindowLength=on  WindowLength=signalWindowLength  SimulateUsing=Code generation
  H : Outport
  L : Outport  Port=2
  wires:
  Moving Minimum/1 -> L/1
  Moving Maximum/1 -> H/1
  IR_ADC/1 -> Moving Minimum/1, Moving Maximum/1

== system MicroMouseTemplate/ADCs /Subsystem1/convert to H and L5 ==
  IR_ADC : Inport
  Moving Maximum : dspstat3/Moving Maximum  SpecifyWindowLength=on  WindowLength=signalWindowLength  SimulateUsing=Code generation
  Moving Minimum : dspstat3/Moving Minimum  SpecifyWindowLength=on  WindowLength=signalWindowLength  SimulateUsing=Code generation
  H : Outport
  L : Outport  Port=2
  wires:
  Moving Minimum/1 -> L/1
  Moving Maximum/1 -> H/1
  IR_ADC/1 -> Moving Minimum/1, Moving Maximum/1

== system MicroMouseTemplate/ADCs /Subsystem1/convert to H and L6 ==
  IR_ADC : Inport
  Moving Maximum : dspstat3/Moving Maximum  SpecifyWindowLength=on  WindowLength=signalWindowLength  SimulateUsing=Code generation
  Moving Minimum : dspstat3/Moving Minimum  SpecifyWindowLength=on  WindowLength=signalWindowLength  SimulateUsing=Code generation
  H : Outport
  L : Outport  Port=2
  wires:
  Moving Minimum/1 -> L/1
  Moving Maximum/1 -> H/1
  IR_ADC/1 -> Moving Minimum/1, Moving Maximum/1

== system MicroMouseTemplate/ADCs /Subsystem1/convert to H and L7 ==
  IR_ADC : Inport
  Moving Maximum1 : dspstat3/Moving Maximum  SpecifyWindowLength=on  WindowLength=signalWindowLength-15  SimulateUsing=Code generation
  Moving Minimum : dspstat3/Moving Minimum  SpecifyWindowLength=on  WindowLength=signalWindowLength  SimulateUsing=Code generation
  Moving Minimum2 : dspstat3/Moving Minimum  SpecifyWindowLength=on  WindowLength=signalWindowLength-5  SimulateUsing=Code generation
  H : Outport
  L : Outport  Port=2
  wires:
  Moving Minimum2/1 -> H/1
  Moving Minimum/1 -> L/1
  IR_ADC/1 -> Moving Maximum1/1, Moving Minimum/1
  Moving Maximum1/1 -> Moving Minimum2/1

== system MicroMouseTemplate/ADCs /Subsystem1/convert to H and L8 ==
  IR_ADC : Inport
  Moving Maximum : dspstat3/Moving Maximum  SpecifyWindowLength=on  WindowLength=signalWindowLength  SimulateUsing=Code generation
  Moving Minimum : dspstat3/Moving Minimum  SpecifyWindowLength=on  WindowLength=signalWindowLength  SimulateUsing=Code generation
  H : Outport
  L : Outport  Port=2
  wires:
  Moving Minimum/1 -> L/1
  Moving Maximum/1 -> H/1
  IR_ADC/1 -> Moving Minimum/1, Moving Maximum/1

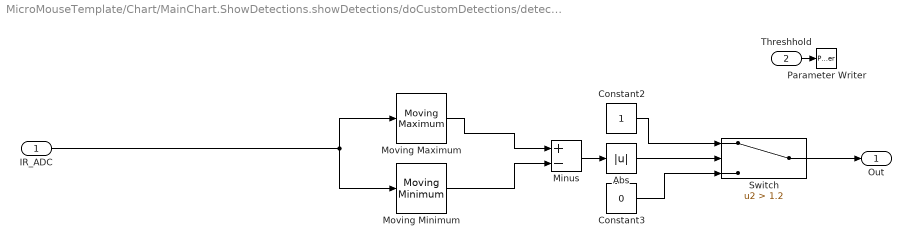
== system MicroMouseTemplate/Chart/MainChart.ShowDetections.showDetections/doCustomDetections/detect_DOWN_LS ==
  IR_ADC : Inport
  Threshhold : Inport  Port=2
  Abs : Abs  SaturateOnIntegerOverflow=off
  Constant2 : Constant
  Constant3 : Constant  Value=0
  Minus : Sum  Inputs=+-  AccumDataTypeStr=single  OutDataTypeStr=single
  Moving Maximum : dspstat3/Moving Maximum  SpecifyWindowLength=on  WindowLength=15  SimulateUsing=Code generation
  Moving Minimum : dspstat3/Moving Minimum  SpecifyWindowLength=on  WindowLength=15  SimulateUsing=Code generation
  Parameter Writer : ParameterWriter  ParameterOwnerBlock=../Switch  ParameterName=Threshold  ParameterInternalName=Threshold
  Switch : Switch  Criteria=u2 > Threshold  Threshold=1.2  SaturateOnIntegerOverflow=off  InputSameDT=off
  Out : Outport
  wires:
  Minus/1 -> Abs/1
  Constant2/1 -> Switch/1
  Moving Minimum/1 -> Minus/2
  Switch/1 -> Out/1
  Constant3/1 -> Switch/3
  Moving Maximum/1 -> Minus/1
  IR_ADC/1 -> Moving Minimum/1, Moving Maximum/1
  Abs/1 -> Switch/2
  Threshhold/1 -> Parameter Writer/1

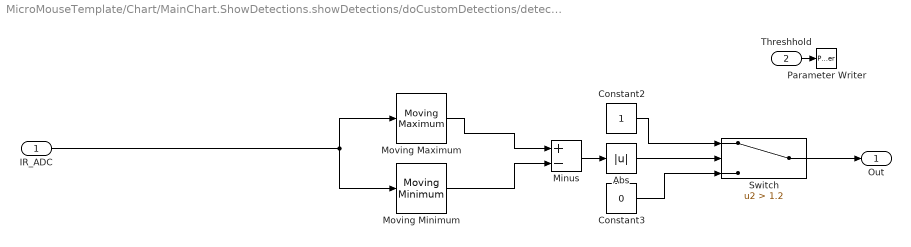
== system MicroMouseTemplate/Chart/MainChart.ShowDetections.showDetections/doCustomDetections/detect_DOWN_RS ==
  IR_ADC : Inport
  Threshhold : Inport  Port=2
  Abs : Abs  SaturateOnIntegerOverflow=off
  Constant2 : Constant
  Constant3 : Constant  Value=0
  Minus : Sum  Inputs=+-  AccumDataTypeStr=single  OutDataTypeStr=single
  Moving Maximum : dspstat3/Moving Maximum  SpecifyWindowLength=on  WindowLength=15  SimulateUsing=Code generation
  Moving Minimum : dspstat3/Moving Minimum  SpecifyWindowLength=on  WindowLength=15  SimulateUsing=Code generation
  Parameter Writer : ParameterWriter  ParameterOwnerBlock=../Switch  ParameterName=Threshold  ParameterInternalName=Threshold
  Switch : Switch  Criteria=u2 > Threshold  Threshold=1.2  SaturateOnIntegerOverflow=off  InputSameDT=off
  Out : Outport
  wires:
  Minus/1 -> Abs/1
  Constant2/1 -> Switch/1
  Moving Minimum/1 -> Minus/2
  Switch/1 -> Out/1
  Constant3/1 -> Switch/3
  Moving Maximum/1 -> Minus/1
  IR_ADC/1 -> Moving Minimum/1, Moving Maximum/1
  Abs/1 -> Switch/2
  Threshhold/1 -> Parameter Writer/1

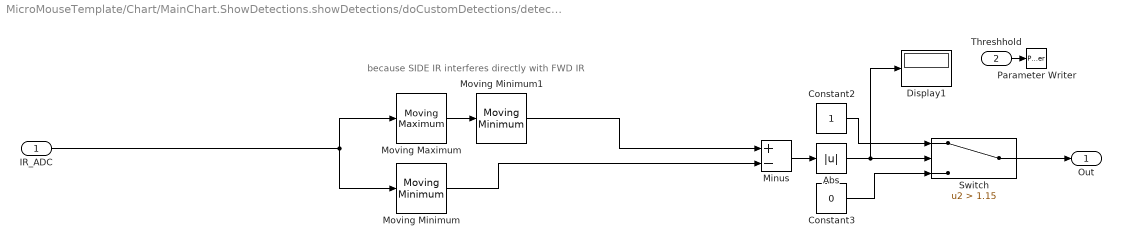
== system MicroMouseTemplate/Chart/MainChart.ShowDetections.showDetections/doCustomDetections/detect_FWD_LS ==
  note: because SIDE IR interferes directly with FWD IR
  IR_ADC : Inport
  Threshhold : Inport  Port=2
  Abs : Abs  SaturateOnIntegerOverflow=off
  Constant2 : Constant
  Constant3 : Constant  Value=0
  Display1 : Display
  Minus : Sum  Inputs=+-  AccumDataTypeStr=single  OutDataTypeStr=single
  Moving Maximum : dspstat3/Moving Maximum  SpecifyWindowLength=on  WindowLength=5  SimulateUsing=Code generation
  Moving Minimum : dspstat3/Moving Minimum  SpecifyWindowLength=on  WindowLength=15  SimulateUsing=Code generation
  Moving Minimum1 : dspstat3/Moving Minimum  SpecifyWindowLength=on  WindowLength=15  SimulateUsing=Code generation
  Parameter Writer : ParameterWriter  ParameterOwnerBlock=../Switch  ParameterName=Threshold  ParameterInternalName=Threshold
  Switch : Switch  Criteria=u2 > Threshold  Threshold=1.15  SaturateOnIntegerOverflow=off  InputSameDT=off
  Out : Outport
  wires:
  Moving Maximum/1 -> Moving Minimum1/1
  Moving Minimum1/1 -> Minus/1
  IR_ADC/1 -> Moving Minimum/1, Moving Maximum/1
  Abs/1 -> Switch/2, Display1/1
  Switch/1 -> Out/1
  Constant3/1 -> Switch/3
  Constant2/1 -> Switch/1
  Minus/1 -> Abs/1
  Threshhold/1 -> Parameter Writer/1
  Moving Minimum/1 -> Minus/2

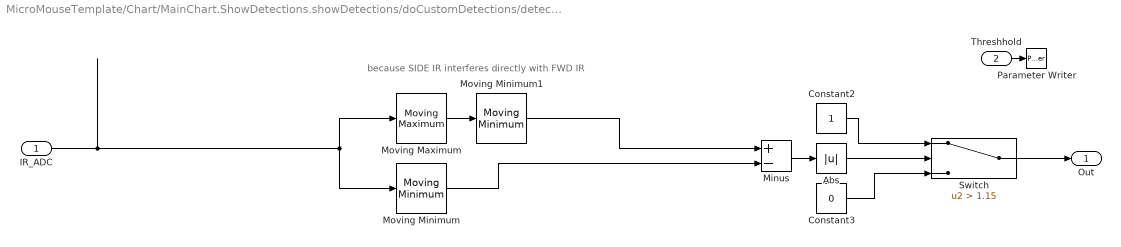
== system MicroMouseTemplate/Chart/MainChart.ShowDetections.showDetections/doCustomDetections/detect_FWD_RS ==
  note: because SIDE IR interferes directly with FWD IR
  IR_ADC : Inport
  Threshhold : Inport  Port=2
  Abs : Abs  SaturateOnIntegerOverflow=off
  Constant2 : Constant
  Constant3 : Constant  Value=0
  Minus : Sum  Inputs=+-  AccumDataTypeStr=single  OutDataTypeStr=single
  Moving Maximum : dspstat3/Moving Maximum  SpecifyWindowLength=on  WindowLength=5  SimulateUsing=Code generation
  Moving Minimum : dspstat3/Moving Minimum  SpecifyWindowLength=on  WindowLength=15  SimulateUsing=Code generation
  Moving Minimum1 : dspstat3/Moving Minimum  SpecifyWindowLength=on  WindowLength=15  SimulateUsing=Code generation
  Parameter Writer : ParameterWriter  ParameterOwnerBlock=../Switch  ParameterName=Threshold  ParameterInternalName=Threshold
  Switch : Switch  Criteria=u2 > Threshold  Threshold=1.15  SaturateOnIntegerOverflow=off  InputSameDT=off
  Out : Outport
  wires:
  Minus/1 -> Abs/1
  Constant2/1 -> Switch/1
  Moving Minimum/1 -> Minus/2
  Switch/1 -> Out/1
  Constant3/1 -> Switch/3
  Moving Maximum/1 -> Moving Minimum1/1
  IR_ADC/1 -> Moving Minimum/1, Moving Maximum/1
  Abs/1 -> Switch/2
  Threshhold/1 -> Parameter Writer/1
  Moving Minimum1/1 -> Minus/1

== system MicroMouseTemplate/Chart/MainChart.ShowDetections.showDetections/doCustomDetections/detect_LS ==
  IR_ADC : Inport
  Threshhold : Inport  Port=2
  Abs : Abs  SaturateOnIntegerOverflow=off
  Constant2 : Constant
  Constant3 : Constant  Value=0
  Minus : Sum  Inputs=+-  AccumDataTypeStr=single  OutDataTypeStr=single
  Moving Maximum : dspstat3/Moving Maximum  SpecifyWindowLength=on  WindowLength=15  SimulateUsing=Code generation
  Moving Minimum : dspstat3/Moving Minimum  SpecifyWindowLength=on  WindowLength=15  SimulateUsing=Code generation
  Parameter Writer : ParameterWriter  ParameterOwnerBlock=../Switch  ParameterName=Threshold  ParameterInternalName=Threshold
  Switch : Switch  Criteria=u2 > Threshold  Threshold=1.2  SaturateOnIntegerOverflow=off  InputSameDT=off
  Out : Outport
  wires:
  Minus/1 -> Abs/1
  Constant2/1 -> Switch/1
  Moving Minimum/1 -> Minus/2
  Switch/1 -> Out/1
  Constant3/1 -> Switch/3
  Moving Maximum/1 -> Minus/1
  IR_ADC/1 -> Moving Minimum/1, Moving Maximum/1
  Abs/1 -> Switch/2
  Threshhold/1 -> Parameter Writer/1

== system MicroMouseTemplate/Chart/MainChart.ShowDetections.showDetections/doCustomDetections/detect_MOT_LS ==
  IR_ADC : Inport
  Threshhold : Inport  Port=2
  Abs : Abs  SaturateOnIntegerOverflow=off
  Constant2 : Constant
  Constant3 : Constant  Value=0
  Minus : Sum  Inputs=+-  AccumDataTypeStr=single  OutDataTypeStr=single
  Moving Maximum : dspstat3/Moving Maximum  SpecifyWindowLength=on  WindowLength=15  SimulateUsing=Code generation
  Moving Minimum : dspstat3/Moving Minimum  SpecifyWindowLength=on  WindowLength=15  SimulateUsing=Code generation
  Parameter Writer : ParameterWriter  ParameterOwnerBlock=../Switch  ParameterName=Threshold  ParameterInternalName=Threshold
  Switch : Switch  Criteria=u2 > Threshold  Threshold=1.2  SaturateOnIntegerOverflow=off  InputSameDT=off
  Out : Outport
  wires:
  Minus/1 -> Abs/1
  Constant2/1 -> Switch/1
  Moving Minimum/1 -> Minus/2
  Switch/1 -> Out/1
  Constant3/1 -> Switch/3
  Moving Maximum/1 -> Minus/1
  IR_ADC/1 -> Moving Minimum/1, Moving Maximum/1
  Abs/1 -> Switch/2
  Threshhold/1 -> Parameter Writer/1

== system MicroMouseTemplate/Chart/MainChart.ShowDetections.showDetections/doCustomDetections/detect_MOT_RS ==
  IR_ADC : Inport
  Threshhold : Inport  Port=2
  Abs : Abs  SaturateOnIntegerOverflow=off
  Constant2 : Constant
  Constant3 : Constant  Value=0
  Minus : Sum  Inputs=+-  AccumDataTypeStr=single  OutDataTypeStr=single
  Moving Maximum : dspstat3/Moving Maximum  SpecifyWindowLength=on  WindowLength=15  SimulateUsing=Code generation
  Moving Minimum : dspstat3/Moving Minimum  SpecifyWindowLength=on  WindowLength=15  SimulateUsing=Code generation
  Parameter Writer : ParameterWriter  ParameterOwnerBlock=../Switch  ParameterName=Threshold  ParameterInternalName=Threshold
  Switch : Switch  Criteria=u2 > Threshold  Threshold=1.2  SaturateOnIntegerOverflow=off  InputSameDT=off
  Out : Outport
  wires:
  Minus/1 -> Abs/1
  Constant2/1 -> Switch/1
  Moving Minimum/1 -> Minus/2
  Switch/1 -> Out/1
  Constant3/1 -> Switch/3
  Moving Maximum/1 -> Minus/1
  IR_ADC/1 -> Moving Minimum/1, Moving Maximum/1
  Abs/1 -> Switch/2
  Threshhold/1 -> Parameter Writer/1

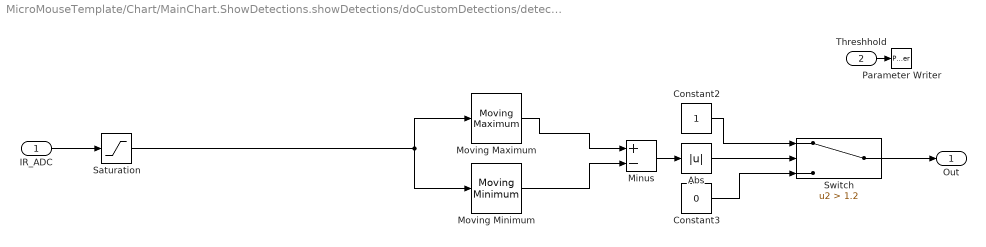
== system MicroMouseTemplate/Chart/MainChart.ShowDetections.showDetections/doCustomDetections/detect_RS ==
  IR_ADC : Inport
  Threshhold : Inport  Port=2
  Abs : Abs  SaturateOnIntegerOverflow=off
  Constant2 : Constant
  Constant3 : Constant  Value=0
  Minus : Sum  Inputs=+-  AccumDataTypeStr=single  OutDataTypeStr=single
  Moving Maximum : dspstat3/Moving Maximum  SpecifyWindowLength=on  WindowLength=15  SimulateUsing=Code generation
  Moving Minimum : dspstat3/Moving Minimum  SpecifyWindowLength=on  WindowLength=15  SimulateUsing=Code generation
  Parameter Writer : ParameterWriter  ParameterOwnerBlock=../Switch  ParameterName=Threshold  ParameterInternalName=Threshold
  Saturation : Saturate  UpperLimit=3.3  LowerLimit=0
  Switch : Switch  Criteria=u2 > Threshold  Threshold=1.2  SaturateOnIntegerOverflow=off  InputSameDT=off
  Out : Outport
  wires:
  Minus/1 -> Abs/1
  Constant2/1 -> Switch/1
  Moving Minimum/1 -> Minus/2
  Switch/1 -> Out/1
  Constant3/1 -> Switch/3
  Moving Maximum/1 -> Minus/1
  IR_ADC/1 -> Saturation/1
  Abs/1 -> Switch/2
  Threshhold/1 -> Parameter Writer/1
  Saturation/1 -> Moving Minimum/1, Moving Maximum/1

== stateflow chart MicroMouseTemplate/Chart ==
  state MainChart
    state Calibrate
      state Cal1
        entry:
        IR_LED_out = [false false false false false false false false];
        during:
        LED0 = ~LED0;
        LED1 = ~LED1;
        LED2 = ~LED2;
        exit:
        LED0 = false;
        LED1 = false;
        LED2 = false;
      state Cal2
        entry:
        vThreshLower = ADC_H - ADC_L;
      state Cal3
        entry:
        IR_LED_out = IR_LED_in;
      state Cal4
        entry:
        vThreshUpper = ADC_H - ADC_L;
        Thresholds = (vThreshUpper + vThreshLower)/2;
        exit:
        LED0 = true;
        LED1 = true;
        LED2 = true;
      (default) -> Cal1
      Cal1 -> Cal2 : [SW1]
      Cal2 -> Cal3 : [SW2]
      Cal3 -> Cal4 : after(1,sec)
    state ShowDetections
      during:
      [LED0,LED1,LED2] = showDetections(ADCs,Thresholds)
      state [LED0,LED1,LED2] = showDetections(ADCs,Thresholds) [function]
    (default) -> Cal2 [order 2] : [SW1]
    (default) -> Calibrate [order 1]
    Cal4 -> ShowDetections : after(1,sec)
  data: LED0 function_output; LED1 function_output; LED2 function_output; ADCs function_input double size=8; Thresholds function_input double size=8; ADCs input double size=8; SW1 input boolean size=1; SW2 input boolean size=1; LED0 output boolean =false; LED1 output boolean =false; LED2 output boolean =false; vThreshLower local double size=8; ADC_H input double size=8; ADC_L input double size=8; IR_LED_out output boolean =[false false false false false false false false];; vThreshUpper local double size=8; IR_LED_in input boolean; Thresholds local double size=8
